simulink model "Simulink_Lotka"  (R2023b)
settings: Solver=ode113  StartTime=0.0  StopTime=20.0  RelTol=1e-9
settings Model: Creator=Filip  LastModifiedBy=Filip

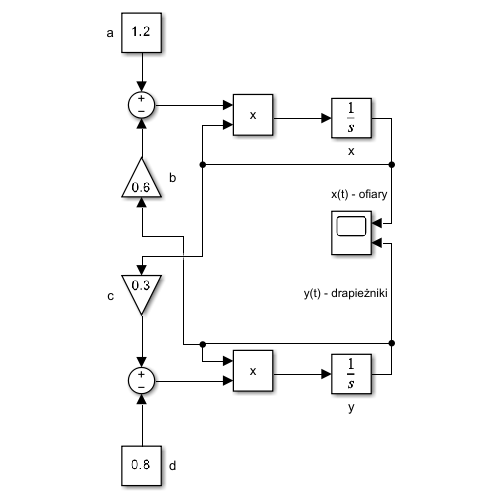
[thumbnail: Simulink's stored preview of the top-level diagram]
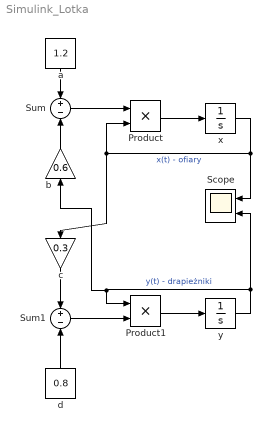
== system Simulink_Lotka ==
  Product : Product
  Product1 : Product
  Scope : Scope  NumInputPorts=2
  Sum : Sum  Inputs=+-
  Sum1 : Sum  Inputs=+-
  a : Constant  Value=1.2
  b : Gain  Gain=0.6
  c : Gain  Gain=0.3
  d : Constant  Value=0.8
  x : Integrator  InitialCondition=2
  y : Integrator  InitialCondition=1
  wires:
  Sum/1 -> Product/1
  Sum1/1 -> Product1/2
  Product1/1 -> y/1
  Product/1 -> x/1
  y/1 -> b/1, Product1/1, Scope/2  "y(t) - drapieżniki"
  d/1 -> Sum1/2
  c/1 -> Sum1/1
  a/1 -> Sum/1
  b/1 -> Sum/2
  x/1 -> Scope/1, c/1, Product/2  "x(t) - ofiary"
